simulink model "U_v1"  (R2016b)
settings: Solver=VariableStepAuto  StartTime=0.0  StopTime=10.0  RelTol=1e-3
settings Model: Creator=黎宇恒  LastModifiedBy=黎宇恒

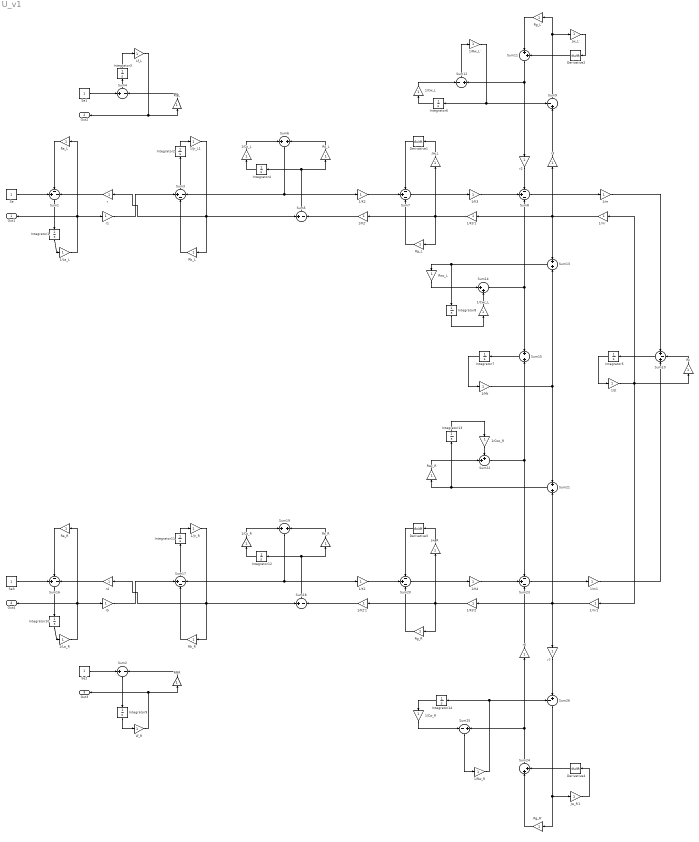
== system U_v1 ==
  1/Cs_L : Gain
  1/Cs_R : Gain
  1/Cw_L : Gain
  1/Cw_R : Gain
  1/Cwc_L : Gain
  1/Cwc_R : Gain
  1/Jr_L1 : Gain
  1/Jr_R : Gain
  1/Jt : Gain
  1/K{1..4} (4 alike) : Gain
  1/K2' : Gain
  1/K2'1 : Gain
  1/K3'1 : Gain
  1/K3'2 : Gain
  1/La_L : Gain
  1/La_R : Gain
  1/Mt : Gain
  1/Rw_L' : Gain
  1/Rw_R : Gain
  1/m : Gain
  1/m' : Gain
  1/m'1 : Gain
  1/m1 : Gain
  Derivative{1..4} (4 alike) : Derivative
  Integrator{1..14} (14 alike) : Integrator
  Jw_L : Gain
  Jw_L' : Gain
  Jw_R : Gain
  Jw_R'1 : Gain
  Lf_L : Gain
  Lf_R : Gain
  Ra_L : Gain
  Ra_R : Gain
  Rb_L : Gain
  Rb_R : Gain
  Rc : Gain
  Rf_L : Gain
  Rf_R : Gain
  Rg_L : Gain
  Rg_L' : Gain
  Rg_R : Gain
  Rg_R' : Gain
  Rs_L : Gain
  Rs_R : Gain
  Rwc_L : Gain
  Rwc_R : Gain
  Se{,1..3} (4 alike) : Constant
  Sum{1,3,16..17} (4 alike) : Sum  Inputs=+--
  Sum10 : Sum  Inputs=+-+
  Sum11 : Sum  Inputs=|++
  Sum12 : Sum  Inputs=-+
  Sum{6,13,15,19,21} (5 alike) : Sum
  Sum14 : Sum  Inputs=|++
  Sum{2,4..5,18} (4 alike) : Sum  Inputs=+-
  Sum{7..8,20,23} (4 alike) : Sum  Inputs=-+-
  Sum22 : Sum  Inputs=++|
  Sum24 : Sum  Inputs=|++
  Sum25 : Sum  Inputs=-+
  Sum26 : Sum  Inputs=-+|
  Sum9 : Sum  Inputs=-+|
  r{,1..7} (8 alike) : Gain
  Out1 : Outport
  Out2 : Outport  Port=2
  Out3 : Outport  Port=3
  Out4 : Outport  Port=4
  wires:
  Se/1 -> Sum1/1
  Ra_L/1 -> Sum1/2
  Sum1/1 -> Integrator1/1
  Integrator1/1 -> 1/La_L/1
  1/La_L/1 -> r1/1, Out1/1, Ra_L/1
  r/1 -> Sum1/3
  r1/1 -> Sum3/1
  Sum3/1 -> Integrator2/1
  Integrator2/1 -> 1/Jr_L1/1
  Rb_L/1 -> Sum3/2
  1/Jr_L1/1 -> Rb_L/1, r/1, Sum5/1
  Sum6/1 -> Sum3/3, 1/K2/1
  Se1/1 -> Sum4/1
  Sum4/1 -> Integrator3/1
  Rf_L/1 -> Sum4/2
  Integrator3/1 -> Lf_L/1
  Lf_L/1 -> Out2/1, Rf_L/1
  1/Cs_L/1 -> Sum6/1
  Integrator4/1 -> 1/Cs_L/1
  Rs_L/1 -> Sum6/2
  Sum5/1 -> Rs_L/1, Integrator4/1
  1/K2'/1 -> Sum5/2
  1/K2/1 -> Sum7/2
  Derivative1/1 -> Sum7/1
  Jw_L/1 -> Derivative1/1
  Sum7/1 -> 1/K3/1
  Rg_L/1 -> Sum7/3
  1/K3'1/1 -> Jw_L/1, Rg_L/1, 1/K2'/1
  1/K3/1 -> Sum8/2
  r2/1 -> Sum8/1
  r3/1 -> Sum9/2
  1/m'/1 -> 1/K3'1/1, Sum13/1, r3/1
  Sum8/1 -> 1/m/1
  Integrator5/1 -> 1/Jt/1
  Sum10/1 -> Integrator5/1
  Rc/1 -> Sum10/2
  1/Jt/1 -> 1/m'1/1, Rc/1, 1/m'/1
  1/m/1 -> Sum10/1
  Sum14/1 -> Sum15/1, Sum8/3
  Sum11/1 -> Sum12/2, r2/1
  Rg_L'/1 -> Sum11/1
  Sum9/1 -> Jw_L'/1, Rg_L'/1
  Derivative2/1 -> Sum11/2
  Jw_L'/1 -> Derivative2/1
  Integrator6/1 -> 1/Cw_L/1
  1/Cw_L/1 -> Sum12/1
  Sum12/1 -> 1/Rw_L'/1
  1/Rw_L'/1 -> Integrator6/1, Sum9/1
  Rwc_L/1 -> Sum14/1
  Sum15/1 -> Integrator7/1
  Integrator7/1 -> 1/Mt/1
  1/Mt/1 -> Sum21/1, Sum13/2
  Sum13/1 -> Rwc_L/1, Integrator8/1
  Integrator8/1 -> 1/Cwc_L/1
  1/Cwc_L/1 -> Sum14/2
  Se2/1 -> Sum2/1
  Sum2/1 -> Integrator9/1
  Rf_R/1 -> Sum2/2
  Integrator9/1 -> Lf_R/1
  Lf_R/1 -> Out3/1, Rf_R/1
  Se3/1 -> Sum16/1
  Ra_R/1 -> Sum16/2
  Sum16/1 -> Integrator10/1
  Integrator10/1 -> 1/La_R/1
  1/La_R/1 -> r5/1, Out4/1, Ra_R/1
  r4/1 -> Sum16/3
  r5/1 -> Sum17/1
  Sum17/1 -> Integrator11/1
  Integrator11/1 -> 1/Jr_R/1
  Rb_R/1 -> Sum17/2
  1/Jr_R/1 -> Rb_R/1, r4/1, Sum18/1
  Sum19/1 -> Sum17/3, 1/K1/1
  1/Cs_R/1 -> Sum19/1
  Integrator12/1 -> 1/Cs_R/1
  Rs_R/1 -> Sum19/2
  Sum18/1 -> Rs_R/1, Integrator12/1
  1/K2'1/1 -> Sum18/2
  1/K1/1 -> Sum20/2
  Derivative3/1 -> Sum20/1
  Jw_R/1 -> Derivative3/1
  Sum20/1 -> 1/K4/1
  Rg_R/1 -> Sum20/3
  1/K3'2/1 -> Jw_R/1, Rg_R/1, 1/K2'1/1
  1/K4/1 -> Sum23/2
  Integrator13/1 -> 1/Cwc_R/1
  Sum21/1 -> Integrator13/1, Rwc_R/1
  1/Cwc_R/1 -> Sum22/1
  Sum22/1 -> Sum23/1, Sum15/2
  Rwc_R/1 -> Sum22/2
  Sum23/1 -> 1/m1/1
  1/m1/1 -> Sum10/3
  r6/1 -> Sum23/3
  1/m'1/1 -> Sum21/2, r7/1, 1/K3'2/1
  Sum24/1 -> Sum25/2, r6/1
  Derivative4/1 -> Sum24/2
  Rg_R'/1 -> Sum24/1
  Sum26/1 -> Rg_R'/1, Jw_R'1/1
  r7/1 -> Sum26/2
  Integrator14/1 -> 1/Cw_R/1
  Sum25/1 -> 1/Rw_R/1
  1/Cw_R/1 -> Sum25/1
  1/Rw_R/1 -> Integrator14/1, Sum26/1
  Jw_R'1/1 -> Derivative4/1
